simulink model "EEPROM_M24C04_Demo"  (R2024b)
settings: Solver=VariableStepAuto  StartTime=0.0  StopTime=2.0  RelTol=1e-3
settings Model: Creator=Shreyas  LastModifiedBy=Shreyas
settings SFSimCC: SimCustomSourceCode="#include \"m24c04.c\""  SimCustomHeaderCode="#include \"m24c04.h\""
settings RTWCC: CustomSourceCode="#include \"m24c04.c\""  CustomHeaderCode="#include \"m24c04.h\""

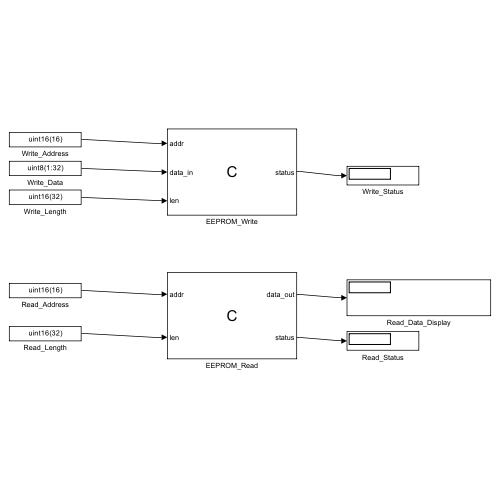
[thumbnail: Simulink's stored preview of the top-level diagram]
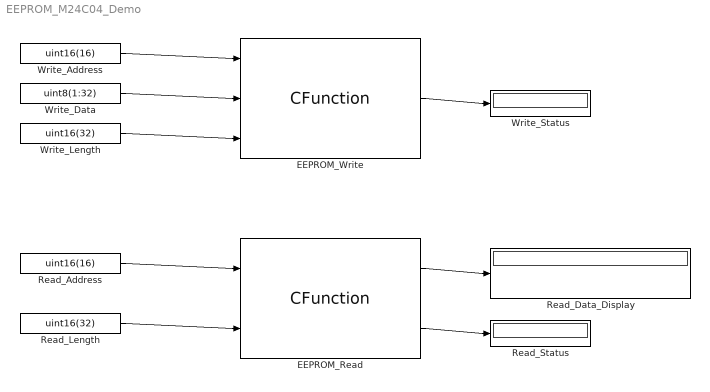
== system EEPROM_M24C04_Demo ==
  EEPROM_Read : CFunction  OutputCode=|  CodegenOutputCode=|  SimCustomHeaderFile=m24c04.h  SimCustomSourceFile=m24c04.c  CustomHeaderFile=m24c04.h  CustomSourceFile=m24c04.c  CustomCodeIsMultiInstantiable=on
      OutputCode=|
      | /* ST M24C04 EEPROM Read Operation */
      | status = M24C04_Read(addr, data_out, len);
      CodegenOutputCode=|
      | /* ST M24C04 EEPROM Read Operation */
      | status = M24C04_Read(addr, data_out, len);
  EEPROM_Write : CFunction  OutputCode=|  CodegenOutputCode=|  SimCustomHeaderFile=m24c04.h  SimCustomSourceFile=m24c04.c  CustomHeaderFile=m24c04.h  CustomSourceFile=m24c04.c  CustomCodeIsMultiInstantiable=on
      OutputCode=|
      | /* ST M24C04 EEPROM Write Operation */
      | status = M24C04_Write(addr, data_in, len);
      CodegenOutputCode=|
      | /* ST M24C04 EEPROM Write Operation */
      | status = M24C04_Write(addr, data_in, len);
  Read_Address : Constant  Value=uint16(16)  OutDataTypeStr=uint16
  Read_Data_Display : Display
  Read_Length : Constant  Value=uint16(32)  OutDataTypeStr=uint16
  Read_Status : Display
  Write_Address : Constant  Value=uint16(16)  OutDataTypeStr=uint16
  Write_Data : Constant  Value=uint8(1:32)  OutDataTypeStr=uint8
  Write_Length : Constant  Value=uint16(32)  OutDataTypeStr=uint16
  Write_Status : Display
  wires:
  Write_Address/1 -> EEPROM_Write/1
  Write_Data/1 -> EEPROM_Write/2
  Write_Length/1 -> EEPROM_Write/3
  EEPROM_Write/1 -> Write_Status/1
  Read_Address/1 -> EEPROM_Read/1
  Read_Length/1 -> EEPROM_Read/2
  EEPROM_Read/1 -> Read_Data_Display/1
  EEPROM_Read/2 -> Read_Status/1
